simulink model "peacockElettricaSimulink"  (R2026a)
settings: Solver=FixedStepAuto  StopTime=40  FixedStep=0.001  EnableMultiTasking=on
InitFcn:
  | run('setupParams.m');
  | %run("tracks\track2.m");
StopFcn:
  | plot(out.X, out.Y);
  | axis equal;
  | grid on;
model workspace: external: MATLAB File (data not in the file)
values from neighbouring files (symbols this model uses):
  aero_bal_r = 0.5    [setupParams.m]    (also in setupParamsSingle.m)
  Af = 1.1    [setupParams.m]    (also in setupParamsSingle.m)
  auto_speed = 0    [setupParams.m]
  ay_limit = 15.0    (= 15)    [setupParams.m]    (also in setupParamsSingle.m)
  brake_bias_f = 0.40    (= 0.4)    [setupParams.m]    (also in setupParamsSingle.m = 0.6)
  brake_bias_r = 1 - brake_bias_f    (= 0.6)    [setupParams.m]    (also in setupParamsSingle.m = 0.4)
  camber_front = -1.5    [setupParams.m]    (also in setupParamsSingle.m)
  camber_rear = -1    [setupParams.m]    (also in setupParamsSingle.m)
  Cl = 1.0    (= 1)    [setupParams.m]    (also in setupParamsSingle.m)
  deathzone_APP = 5    [setupParams.m]    (also in setupParamsSingle.m)
  e_yaw_deadzone = 0.03    [setupParams.m]
  falling_slew_rate_torque = -500    [setupParams.m]    (also in setupParamsSingle.m)
  g = 9.81    [setupParams.m]    (also in setupParamsSingle.m)
  gnd_displ = 0.0    (= 0)    [setupParams.m]    (also in setupParamsSingle.m)
  h_o = 0.35    [setupParams.m]    (also in setupParamsSingle.m)
  I_charge_max = 21    [setupParams.m]
  I_discharge_max = 90    [setupParams.m]
  K_roll_rear = 0.6    [setupParams.m]    (also in setupParamsSingle.m = 0.5)
  Kus = 0.03    [setupParams.m]    (also in setupParamsSingle.m = 0)
  l_f = 0.775    [setupParams.m]    (also in setupParamsSingle.m)
  l_r = 0.775    [setupParams.m]    (also in setupParamsSingle.m)
  launch_ramp_rate = 1000.0    (= 1000)    [setupParams.m]    (also in setupParamsSingle.m)
  launch_V_thresh = 5.0    (= 5)    [setupParams.m]    (also in setupParamsSingle.m)
  mass = 320    [setupParams.m]    (also in setupParamsSingle.m = 300)
  mu = 1.5    [setupParams.m]    (also in setupParamsSingle.m)
  nominal_ramp_rate = 1000.0    (= 1000)    [setupParams.m]    (also in setupParamsSingle.m)
  overslip_factor = 1.01    [setupParams.m]    (also in setupParamsSingle.m = 1.13)
  pa_front_wheel = 82700    [setupParams.m]    (also in setupParamsSingle.m)
  pa_rear_wheel = 82700    [setupParams.m]    (also in setupParamsSingle.m)
  pedal_bp = (0:10:100)'    [setupParams.m]    (also in setupParamsSingle.m)
  pedal_map = (pedal_bp / 100) .^ pedal_alpha    [setupParams.m]    (also in setupParamsSingle.m = (pedal_bp / 100) .^ pedal_alpha.Value)
  R_wheel = 0.2032    [setupParams.m]    (also in setupParamsSingle.m)
  regen_I_cont_A = 14.0    (= 14)    [setupParams.m]    (also in setupParamsSingle.m)
  regen_I_peak_A = 21.0    (= 21)    [setupParams.m]    (also in setupParamsSingle.m)
  regen_I_peak_dur_s = 4.0    (= 4)    [setupParams.m]    (also in setupParamsSingle.m)
  regen_P_batt_max_W = 35000    [setupParams.m]    (also in setupParamsSingle.m)
  regen_pedal_thr = 5.0    (= 5)    [setupParams.m]    (also in setupParamsSingle.m = 10)
  regen_speed_crit_rpm = 1000    [setupParams.m]    (also in setupParamsSingle.m = 500)
  regen_speed_min_rpm = 4000    [setupParams.m]    (also in setupParamsSingle.m = 3000)
  regen_T_max = 9    [setupParams.m]    (also in setupParamsSingle.m = Simulink.Parameter(T_rated.Value/2))
  rho = 1.225    [setupParams.m]    (also in setupParamsSingle.m)
  rid_eff = 0.80    (= 0.8)    [setupParams.m]    (also in setupParamsSingle.m)
  rid_ratio = 15    [setupParams.m]    (also in setupParamsSingle.m)
  rising_slew_rate_torque = 100    [setupParams.m]    (also in setupParamsSingle.m)
  rpm_safe_threshold = 100    [setupParams.m]
  scale_factor_front = ones(27, 1)    [setupParams.m]    (also in setupParamsSingle.m)
  scale_factor_rear = ones(27, 1)    [setupParams.m]    (also in setupParamsSingle.m)
  slip_bc_coeff = 10    [setupParams.m]    (also in setupParamsSingle.m = Simulink.Parameter(1.5))
  slip_filt_N = 80    [setupParams.m]    (also in setupParamsSingle.m = 15)
  slip_Kd = 0.8    [setupParams.m]    (also in setupParamsSingle.m = Simulink.Parameter(5.0))
  slip_Ki = 13.0    (= 13)    [setupParams.m]    (also in setupParamsSingle.m = Simulink.Parameter(110.0))
  slip_Kp = 50.0    (= 50)    [setupParams.m]    (also in setupParamsSingle.m = Simulink.Parameter(180.0))
  slip_low_sat = 0.0    (= 0)    [setupParams.m]    (also in setupParamsSingle.m)
  slip_ref = 0.15    [setupParams.m]    (also in setupParamsSingle.m = Simulink.Parameter(0.15))
  slip_up_sat = 25    [setupParams.m]    (also in setupParamsSingle.m = 21)
  slip_V_min = 3    [setupParams.m]    (also in setupParamsSingle.m = 1)
  steer_ratio = 4.2    [pure_pursuit.m]    (also in setupParams.m; setupParamsSingle.m)
  steering_deadband = 1    [setupParams.m]
  T_headroom_k = 13.0    (= 13)    [setupParams.m]    (also in setupParamsSingle.m = Simulink.Parameter(5.0))
  T_headroom_max = 9    [setupParams.m]    (also in setupParamsSingle.m = Simulink.Parameter(5.0))
  T_peak = 20    [setupParams.m]    (also in setupParamsSingle.m = 21)
  T_rated = 9.8    [setupParams.m]    (also in setupParamsSingle.m = Simulink.Parameter(9.8))
  track_width = (track_width_r + track_width_f)/2    (= 1.2)    [setupParams.m]    (also in setupParamsSingle.m = sqrt(track_width_r^2 + track_width_f^2))
  track_width_f = 1.2    [setupParams.m]    (also in setupParamsSingle.m)
  track_width_r = 1.2    [setupParams.m]    (also in setupParamsSingle.m)
  Ts = 0.01    [setupParams.m]    (also in setupParamsSingle.m)
  tvc_bc = 17    [setupParams.m]
  tvc_D_thresh = 0.060    (= 0.06)    [setupParams.m]    (also in setupParamsSingle.m)
  tvc_D_thresh_off = 0.03    [setupParams.m]    (also in setupParamsSingle.m)
  tvc_Kd = 100    [setupParams.m]    (also in setupParamsSingle.m = Simulink.Parameter(5))
  tvc_Ki = 150    [setupParams.m]    (also in setupParamsSingle.m = Simulink.Parameter(10))
  tvc_Kp = 650    [setupParams.m]    (also in setupParamsSingle.m = Simulink.Parameter(70))
  tvc_N_filter = 25    [setupParams.m]    (also in setupParamsSingle.m = Simulink.Parameter(20))
  tvc_sat_dMz = 700    [setupParams.m]    (also in setupParamsSingle.m = Simulink.Parameter(10.0))
  tvc_throttle_on = 3.0    (= 3)    [setupParams.m]    (also in setupParamsSingle.m = Simulink.Parameter(3.0))
  tvc_tr = 5    [setupParams.m]    (also in setupParamsSingle.m = Simulink.Parameter(1.0))
  tvc_V_off = 2.0    (= 2)    [setupParams.m]    (also in setupParamsSingle.m = Simulink.Parameter(2.0))
  tvc_V_on = 4.0    (= 4)    [setupParams.m]    (also in setupParamsSingle.m = Simulink.Parameter(4.0))
  tvc_yaw_thresh = 0.08    [setupParams.m]    (also in setupParamsSingle.m)
  tvc_yaw_thresh_off = 0.04    [setupParams.m]    (also in setupParamsSingle.m)
  V_dc = 540    [setupParams.m]    (also in setupParamsSingle.m)
  w_engine = 0.005    [setupParams.m]    (also in setupParamsSingle.m)
  wheelbase = l_f + l_r    (= 1.55)    [setupParams.m]    (also in setupParamsSingle.m)
undefined symbols (not defined in the file or in its folder): V_ref, X_ref, Y_ref
libraries: simulink x74, slpidlib x8, vehdynlibtire x8, dspsigops x4, vehdynlibsteering x2, autolibshared x2, sim3dautolib x2, sim3dlib x1, robotalgslib x1
(part 4 of 6)

== system peacockElettricaSimulink/DriveController_/MTFC ==
  note: Minimum Torque Follower Controller
      | (derating)
  Throttle : Inport
  Derating_RL : Inport  Port=2
  Derating_RR : Inport  Port=3
  Constant : Constant  Value=T_peak
  Constant1 : Constant  Value=T_rated
  Gain : Gain  Gain=T_peak*0.01
  Logical Operator : Logic  Operator=OR  AllPortsSameDT=off  OutDataTypeStr=boolean
  Min : MinMax  Inputs=2
  Rate Limiter : RateLimiter  RisingSlewLimit=250  FallingSlewLimit=-250  SampleTimeMode=inherited
  Rate Limiter1 : RateLimiter  RisingSlewLimit=250  FallingSlewLimit=-10  SampleTimeMode=inherited
  Switch : Switch  Criteria=u2 > Threshold  Threshold=0.5  SaturateOnIntegerOverflow=off  InputSameDT=off
  T_req_MTFC : Outport
  wires:
  Min/1 -> Rate Limiter1/1  "out"
  Derating_RL/1 -> Logical Operator/1
  Logical Operator/1 -> Switch/2  "or"
  Derating_RR/1 -> Logical Operator/2
  Throttle/1 -> Gain/1
  Constant1/1 -> Switch/1  "rated"
  Constant/1 -> Switch/3  "peak"
  Switch/1 -> Rate Limiter/1
  Gain/1 -> Min/1  "req"
  Rate Limiter/1 -> Min/2  "T_lim_HW"
  Rate Limiter1/1 -> T_req_MTFC/1  "T_lim_HW"

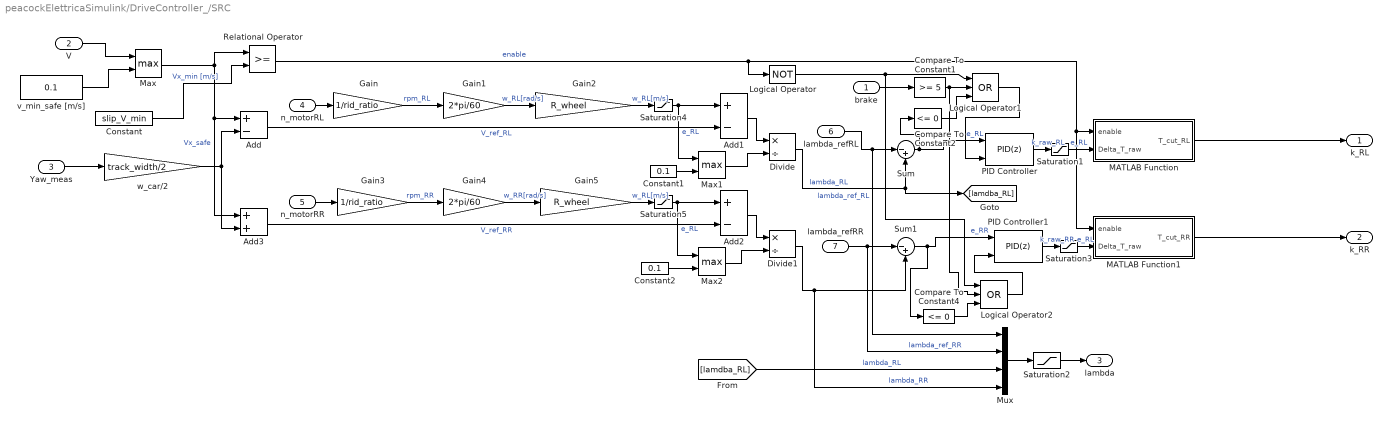
== system peacockElettricaSimulink/DriveController_/SRC ==
  brake : Inport
  V : Inport  Port=2
  Yaw_meas : Inport  Port=3
  n_motorRL : Inport  Port=4
  n_motorRR : Inport  Port=5
  lambda_refRL : Inport  Port=6
  lambda_refRR : Inport  Port=7
  Add : Sum  Inputs=+-
  Add1 : Sum  Inputs=+-
  Add2 : Sum  Inputs=+-
  Add3 : Sum
  Compare To Constant1 : simulink/Logic and Bit Operations/Compare To Constant  relop=>=  const=5  OutDataTypeStr=boolean
  Compare To Constant2 : simulink/Logic and Bit Operations/Compare To Constant  relop=<=  const=0  OutDataTypeStr=boolean
  Compare To Constant4 : simulink/Logic and Bit Operations/Compare To Constant  relop=<=  const=0  OutDataTypeStr=boolean
  Constant : Constant  Value=slip_V_min
  Constant1 : Constant  Value=0.1
  Constant2 : Constant  Value=0.1
  Divide : Product  Inputs=*/
  Divide1 : Product  Inputs=*/
  Gain : Gain  Gain=1/rid_ratio
  Gain1 : Gain  Gain=2*pi/60
  Gain2 : Gain  Gain=R_wheel
  Gain3 : Gain  Gain=1/rid_ratio
  Gain4 : Gain  Gain=2*pi/60
  Gain5 : Gain  Gain=R_wheel
  Logical Operator : Logic  Operator=NOT  AllPortsSameDT=off  OutDataTypeStr=boolean
  Logical Operator1 : Logic  Operator=OR  Inputs=3  AllPortsSameDT=off  OutDataTypeStr=boolean
  Logical Operator2 : Logic  Operator=OR  Inputs=3  AllPortsSameDT=off  OutDataTypeStr=boolean
  MATLAB Function : MATLAB Function  TreatAsAtomicUnit=on
  MATLAB Function1 : MATLAB Function  TreatAsAtomicUnit=on
  Max : MinMax  Function=max  Inputs=2
  Max1 : MinMax  Function=max  Inputs=2
  Max2 : MinMax  Function=max  Inputs=2
  Mux : Mux
  PID Controller : slpidlib/PID Controller  Controller=PID  Form=Parallel  TimeDomain=Discrete-time  UseExternalTs=off  SampleTime=Ts  IntegratorMethod=Forward Euler  FilterMethod=Forward Euler  ControllerParametersSource=internal  P=slip_Kp  I=slip_Ki  UseKiTs=off  D=slip_Kd  UseExternalDerivativeSource=off  N=slip_filt_N  UseFilter=on  TunerSelectOption=Transfer Function Based (PID Tuner App)  InitialConditionSource=internal  InitialConditionForIntegrator=0  InitialConditionForFilter=0  DifferentiatorICPrevScaledInput=0  ExternalReset=level  TrackingMode=off  Kt=1  LimitOutput=on  SatLimitsSource=internal  UpperSaturationLimit=slip_up_sat  LowerSaturationLimit=slip_low_sat  LinearizeAsGain=on  AntiWindupMode=back-calculation  Kb=slip_bc_coeff  LimitIntegrator=on  UpperIntegratorSaturationLimit=slip_up_sat  LowerIntegratorSaturationLimit=slip_low_sat  POutMin=[]  POutMax=[]  IOutMin=[]  IOutMax=[]  DOutMin=[]  DOutMax=[]  NOutMin=[]  NOutMax=[]  SumOutMin=[]  SumOutMax=[]  SaturationOutMin=[]  SaturationOutMax=[]  PParamMin=[]  PParamMax=[]  IParamMin=[]  IParamMax=[]  DParamMin=[]  DParamMax=[]  NParamMin=[]  NParamMax=[]  KbParamMin=[]  KbParamMax=[]  KtParamMin=[]  KtParamMax=[]  KbOutMin=[]  KbOutMax=[]  KtOutMin=[]  KtOutMax=[]  IntegratorOutMin=[]  IntegratorOutMax=[]  FilterOutMin=[]  FilterOutMax=[]  SumI1OutMin=[]  SumI1OutMax=[]  SumI2OutMin=[]  SumI2OutMax=[]  SumI3OutMin=[]  SumI3OutMax=[]  SumI4OutMin=[]  SumI4OutMax=[]  SumDOutMin=[]  SumDOutMax=[]  DifferentiatorOutMin=[]  DifferentiatorOutMax=[]  FilterDiffOutCoefMin=[]  FilterDiffOutCoefMax=[]  ReciprocalOutMin=[]  ReciprocalOutMax=[]  SumDenOutMin=[]  SumDenOutMax=[]  SumNumOutMin=[]  SumNumOutMax=[]  DivideOutMin=[]  DivideOutMax=[]  UdiffTsProdOutMin=[]  UdiffTsProdOutMax=[]  NTsProdOutMin=[]  NTsProdOutMax=[]  UintegralTsProdOutMin=[]  UintegralTsProdOutMax=[]  UngainTsProdOutMin=[]  UngainTsProdOutMax=[]  ClampingZeroOutDataTypeStr=Inherit: Inherit via back propagation  ClampingZeroOutMin=[]  ClampingZeroOutMax=[]  FilterDenConstantOutDataTypeStr=Inherit: Inherit via back propagation  FilterDenConstantOutMin=[]  FilterDenConstantOutMax=[]  PCopyOutDataTypeStr=Inherit: Inherit via back propagation  PCopyOutMin=[]  PCopyOutMax=[]  NCopyOutDataTypeStr=Inherit: Inherit via back propagation  NCopyOutMin=[]  NCopyOutMax=[]  IntegratorContinuousStateAttributes=''  IntegratorStateMustResolveToSignalObject=off  IntegratorRTWStateStorageClass=Auto  FilterContinuousStateAttributes=''  FilterStateMustResolveToSignalObject=off  FilterRTWStateStorageClass=Auto  ParallelPVariant=InternalParameters  IdealPVariant=Disabled  IVariant=InternalParameters  DVariant=InternalParameters  IntegratorVariant=Discrete  SatVariant=Enabled  AWVariant=BackCalculation  PCopyVariant=Disabled  TRVariant=Disabled  FdbkBlocksVariant=Forward  IdealPFdbkVariant=Disabled  SatFdbkVariant=Disabled  DerivativeFilterVariant=ForwardEulerFilter  NVariant=InternalParameters  NCopyVariant=Disabled  FilterICVariant=InternalICsFilter  IntegratorICVariant=InternalICs  ExternalResetVariant=ExternalReset  TRSumVariant=Passthrough  SumFdbkVariant=Disabled  SumVariant=Sum_PID  TsampFilterVariant=InternalTs  TsampNgainVariant=Passthrough  TsampIntegralVariant=Disabled_SignalSpec  ExternalSaturationOutDataTypeStr=Inherit: Same as second input  DerivativeSourceVariant=ErrorSignal  PreIntVariant=InternalPreInt
  PID Controller1 : slpidlib/PID Controller  Controller=PID  Form=Parallel  TimeDomain=Discrete-time  UseExternalTs=off  SampleTime=Ts  IntegratorMethod=Forward Euler  FilterMethod=Forward Euler  ControllerParametersSource=internal  P=slip_Kp  I=slip_Ki  UseKiTs=off  D=slip_Kd  UseExternalDerivativeSource=off  N=slip_filt_N  UseFilter=on  TunerSelectOption=Transfer Function Based (PID Tuner App)  InitialConditionSource=internal  InitialConditionForIntegrator=0  InitialConditionForFilter=0  DifferentiatorICPrevScaledInput=0  ExternalReset=level  TrackingMode=off  Kt=1  LimitOutput=on  SatLimitsSource=internal  UpperSaturationLimit=slip_up_sat  LowerSaturationLimit=slip_low_sat  LinearizeAsGain=on  AntiWindupMode=back-calculation  Kb=slip_bc_coeff  LimitIntegrator=on  UpperIntegratorSaturationLimit=slip_up_sat  LowerIntegratorSaturationLimit=slip_low_sat  POutMin=[]  POutMax=[]  IOutMin=[]  IOutMax=[]  DOutMin=[]  DOutMax=[]  NOutMin=[]  NOutMax=[]  SumOutMin=[]  SumOutMax=[]  SaturationOutMin=[]  SaturationOutMax=[]  PParamMin=[]  PParamMax=[]  IParamMin=[]  IParamMax=[]  DParamMin=[]  DParamMax=[]  NParamMin=[]  NParamMax=[]  KbParamMin=[]  KbParamMax=[]  KtParamMin=[]  KtParamMax=[]  KbOutMin=[]  KbOutMax=[]  KtOutMin=[]  KtOutMax=[]  IntegratorOutMin=[]  IntegratorOutMax=[]  FilterOutMin=[]  FilterOutMax=[]  SumI1OutMin=[]  SumI1OutMax=[]  SumI2OutMin=[]  SumI2OutMax=[]  SumI3OutMin=[]  SumI3OutMax=[]  SumI4OutMin=[]  SumI4OutMax=[]  SumDOutMin=[]  SumDOutMax=[]  DifferentiatorOutMin=[]  DifferentiatorOutMax=[]  FilterDiffOutCoefMin=[]  FilterDiffOutCoefMax=[]  ReciprocalOutMin=[]  ReciprocalOutMax=[]  SumDenOutMin=[]  SumDenOutMax=[]  SumNumOutMin=[]  SumNumOutMax=[]  DivideOutMin=[]  DivideOutMax=[]  UdiffTsProdOutMin=[]  UdiffTsProdOutMax=[]  NTsProdOutMin=[]  NTsProdOutMax=[]  UintegralTsProdOutMin=[]  UintegralTsProdOutMax=[]  UngainTsProdOutMin=[]  UngainTsProdOutMax=[]  ClampingZeroOutDataTypeStr=Inherit: Inherit via back propagation  ClampingZeroOutMin=[]  ClampingZeroOutMax=[]  FilterDenConstantOutDataTypeStr=Inherit: Inherit via back propagation  FilterDenConstantOutMin=[]  FilterDenConstantOutMax=[]  PCopyOutDataTypeStr=Inherit: Inherit via back propagation  PCopyOutMin=[]  PCopyOutMax=[]  NCopyOutDataTypeStr=Inherit: Inherit via back propagation  NCopyOutMin=[]  NCopyOutMax=[]  IntegratorContinuousStateAttributes=''  IntegratorStateMustResolveToSignalObject=off  IntegratorRTWStateStorageClass=Auto  FilterContinuousStateAttributes=''  FilterStateMustResolveToSignalObject=off  FilterRTWStateStorageClass=Auto  ParallelPVariant=InternalParameters  IdealPVariant=Disabled  IVariant=InternalParameters  DVariant=InternalParameters  IntegratorVariant=Discrete  SatVariant=Enabled  AWVariant=BackCalculation  PCopyVariant=Disabled  TRVariant=Disabled  FdbkBlocksVariant=Forward  IdealPFdbkVariant=Disabled  SatFdbkVariant=Disabled  DerivativeFilterVariant=ForwardEulerFilter  NVariant=InternalParameters  NCopyVariant=Disabled  FilterICVariant=InternalICsFilter  IntegratorICVariant=InternalICs  ExternalResetVariant=ExternalReset  TRSumVariant=Passthrough  SumFdbkVariant=Disabled  SumVariant=Sum_PID  TsampFilterVariant=InternalTs  TsampNgainVariant=Passthrough  TsampIntegralVariant=Disabled_SignalSpec  ExternalSaturationOutDataTypeStr=Inherit: Same as second input  DerivativeSourceVariant=ErrorSignal  PreIntVariant=InternalPreInt
  Relational Operator : RelationalOperator  OutDataTypeStr=boolean  RndMeth=Simplest  InputSameDT=off
  Saturation1 : Saturate  UpperLimit=inf  LowerLimit=-2
  Saturation2 : Saturate  UpperLimit=1  LowerLimit=0
  Saturation3 : Saturate  UpperLimit=inf  LowerLimit=-2
  Saturation4 : Saturate  UpperLimit=inf  LowerLimit=0
  Saturation5 : Saturate  UpperLimit=inf  LowerLimit=0
  Sum : Sum  Inputs=|-+
  Sum1 : Sum  Inputs=|-+
  v_min_safe [m/s] : Constant  Value=0.1
  w_car/2 : Gain  Gain=track_width/2
  k_RL : Outport
  k_RR : Outport  Port=2
  lambda : Outport  Port=3
  wires:
  V/1 -> Max/1
  v_min_safe [m/s]/1 -> Max/2
  Max/1 -> Relational Operator/1, Add3/1, Add/1  "Vx_safe"
  Constant/1 -> Relational Operator/2  "Vx_min [m/s]"
  Yaw_meas/1 -> w_car/2/1
  Add/1 -> Add1/2  "V_ref_RL"
  n_motorRL/1 -> Gain/1
  Gain/1 -> Gain1/1  "rpm_RL"
  Add1/1 -> Divide/1
  Divide/1 -> [lamdba_RL], Sum/2  "lambda_RL"
  w_car/2/1 -> Add3/2, Add/2
  Gain1/1 -> Gain2/1  "w_RL[rad/s]"
  Gain2/1 -> Saturation4/1  "w_RL[m/s]"
  Gain4/1 -> Gain5/1  "w_RR[rad/s]"
  Gain3/1 -> Gain4/1  "rpm_RR"
  Divide1/1 -> Sum1/2, Mux/4  "lambda_RR"
  n_motorRR/1 -> Gain3/1
  Add3/1 -> Add2/2  "V_ref_RR"
  Add2/1 -> Divide1/1
  Relational Operator/1 -> MATLAB Function1/1(enable), MATLAB Function/1(enable), Logical Operator/1  "enable"
  PID Controller/1 -> Saturation1/1  "k_raw_RL"
  MATLAB Function/1(T_cut_RL) -> k_RL/1
  PID Controller1/1 -> Saturation3/1  "k_raw_RR"
  lambda_refRR/1 -> Mux/2, Sum1/1  "lambda_ref_RR"
  MATLAB Function1/1(T_cut_RR) -> k_RR/1
  Sum1/1 -> Compare To Constant4/1, PID Controller1/1  "e_RR"
  Sum/1 -> PID Controller/1, Compare To Constant2/1  "e_RL"
  Max1/1 -> Divide/2
  Constant1/1 -> Max1/2
  Max2/1 -> Divide1/2
  Constant2/1 -> Max2/2
  Gain5/1 -> Saturation5/1  "w_RL[m/s]"
  Mux/1 -> Saturation2/1
  Saturation2/1 -> lambda/1
  Saturation1/1 -> MATLAB Function/2(Delta_T_raw)  "e_RL"
  Saturation3/1 -> MATLAB Function1/2(Delta_T_raw)  "e_RL"
  Logical Operator1/1 -> PID Controller/2
  [lamdba_RL] -> Mux/3  "lambda_RL"
  Saturation4/1 -> Max1/1, Add1/1  "e_RL"
  Saturation5/1 -> Max2/1, Add2/1  "e_RL"
  Logical Operator/1 -> Logical Operator2/1, Logical Operator1/1
  Compare To Constant2/1 -> Logical Operator1/3
  Compare To Constant4/1 -> Logical Operator2/3
  lambda_refRL/1 -> Mux/1, Sum/1  "lambda_ref_RL"
  Logical Operator2/1 -> PID Controller1/2
  brake/1 -> Compare To Constant1/1
  Compare To Constant1/1 -> Logical Operator2/2, Logical Operator1/2

== system peacockElettricaSimulink/DriveController_/TVC ==
  note: Momento Imbardata di correzione
  T_req : Inport
  e_yaw : Inport  Port=2
  T_RL_act : Inport  Port=3
  T_RR_act : Inport  Port=4
  n_motorRL : Inport  Port=5
  n_motorRR : Inport  Port=6
  D : Inport  Port=7
  w_slip : Inport  Port=8
  T_max_RL : Inport  Port=9
  T_max_RR : Inport  Port=10
  1-D Lookup Table : Lookup_n-D  NumberOfTableDimensions=1  BreakpointsForDimension1=[0,steering_deadband,5]  Table=[0,0,1]  ExtrapMethod=Clip  UseLastTableValue=on  InternalRulePriority=Speed  RndMeth=Simplest
  Abs1 : Abs  SaturateOnIntegerOverflow=off
  Compare To Constant3 : simulink/Logic and Bit Operations/Compare To Constant  relop===  const=0  OutDataTypeStr=boolean
  Constant : Constant  Value=0
  Dead Zone : DeadZone  LowerValue=-e_yaw_deadzone  UpperValue=e_yaw_deadzone
  Gain : Gain  Gain=180*steer_ratio/pi
  MATLAB Function : MATLAB Function  TreatAsAtomicUnit=on
  MATLAB Function1 : MATLAB Function  TreatAsAtomicUnit=on
  Memory : Memory
  PID Controller : slpidlib/PID Controller  Controller=PID  Form=Parallel  TimeDomain=Discrete-time  UseExternalTs=off  SampleTime=Ts  IntegratorMethod=Forward Euler  FilterMethod=Forward Euler  ControllerParametersSource=internal  P=tvc_Kp  I=tvc_Ki  UseKiTs=off  D=tvc_Kd  UseExternalDerivativeSource=off  N=tvc_N_filter  UseFilter=on  TunerSelectOption=Transfer Function Based (PID Tuner App)  InitialConditionSource=external  InitialConditionForIntegrator=0  InitialConditionForFilter=0  DifferentiatorICPrevScaledInput=0  ExternalReset=level  TrackingMode=on  Kt=tvc_tr  LimitOutput=on  SatLimitsSource=internal  UpperSaturationLimit=tvc_sat_dMz  LowerSaturationLimit=-tvc_sat_dMz  LinearizeAsGain=on  AntiWindupMode=back-calculation  Kb=tvc_bc  LimitIntegrator=off  UpperIntegratorSaturationLimit=inf  LowerIntegratorSaturationLimit=-inf  POutMin=[]  POutMax=[]  IOutMin=[]  IOutMax=[]  DOutMin=[]  DOutMax=[]  NOutMin=[]  NOutMax=[]  SumOutMin=[]  SumOutMax=[]  SaturationOutMin=[]  SaturationOutMax=[]  PParamMin=[]  PParamMax=[]  IParamMin=[]  IParamMax=[]  DParamMin=[]  DParamMax=[]  NParamMin=[]  NParamMax=[]  KbParamMin=[]  KbParamMax=[]  KtParamMin=[]  KtParamMax=[]  KbOutMin=[]  KbOutMax=[]  KtOutMin=[]  KtOutMax=[]  IntegratorOutMin=[]  IntegratorOutMax=[]  FilterOutMin=[]  FilterOutMax=[]  SumI1OutMin=[]  SumI1OutMax=[]  SumI2OutMin=[]  SumI2OutMax=[]  SumI3OutMin=[]  SumI3OutMax=[]  SumI4OutMin=[]  SumI4OutMax=[]  SumDOutMin=[]  SumDOutMax=[]  DifferentiatorOutMin=[]  DifferentiatorOutMax=[]  FilterDiffOutCoefMin=[]  FilterDiffOutCoefMax=[]  ReciprocalOutMin=[]  ReciprocalOutMax=[]  SumDenOutMin=[]  SumDenOutMax=[]  SumNumOutMin=[]  SumNumOutMax=[]  DivideOutMin=[]  DivideOutMax=[]  UdiffTsProdOutMin=[]  UdiffTsProdOutMax=[]  NTsProdOutMin=[]  NTsProdOutMax=[]  UintegralTsProdOutMin=[]  UintegralTsProdOutMax=[]  UngainTsProdOutMin=[]  UngainTsProdOutMax=[]  ClampingZeroOutDataTypeStr=Inherit: Inherit via back propagation  ClampingZeroOutMin=[]  ClampingZeroOutMax=[]  FilterDenConstantOutDataTypeStr=Inherit: Inherit via back propagation  FilterDenConstantOutMin=[]  FilterDenConstantOutMax=[]  PCopyOutDataTypeStr=Inherit: Inherit via back propagation  PCopyOutMin=[]  PCopyOutMax=[]  NCopyOutDataTypeStr=Inherit: Inherit via back propagation  NCopyOutMin=[]  NCopyOutMax=[]  IntegratorContinuousStateAttributes=''  IntegratorStateMustResolveToSignalObject=off  IntegratorRTWStateStorageClass=Auto  FilterContinuousStateAttributes=''  FilterStateMustResolveToSignalObject=off  FilterRTWStateStorageClass=Auto  ParallelPVariant=InternalParameters  IdealPVariant=Disabled  IVariant=InternalParameters  DVariant=InternalParameters  IntegratorVariant=Discrete  SatVariant=Enabled  AWVariant=BackCalculation  PCopyVariant=Disabled  TRVariant=Enabled  FdbkBlocksVariant=Forward  IdealPFdbkVariant=Disabled  SatFdbkVariant=Disabled  DerivativeFilterVariant=ForwardEulerFilter  NVariant=InternalParameters  NCopyVariant=Disabled  FilterICVariant=ExternalICs  IntegratorICVariant=ExternalICs  ExternalResetVariant=ExternalReset  TRSumVariant=TrackingMode  SumFdbkVariant=Disabled  SumVariant=Sum_PID  TsampFilterVariant=InternalTs  TsampNgainVariant=Passthrough  TsampIntegralVariant=Disabled_SignalSpec  ExternalSaturationOutDataTypeStr=Inherit: Same as second input  DerivativeSourceVariant=ErrorSignal  PreIntVariant=InternalPreInt
  Product : Product  Inputs=3
  Scope : Scope  NumInputPorts=3
      settings: ActiveDisplayYMinimum=-0.17006762266637193  ActiveDisplayYMaximum=0.69301535210007792
  Sum3 : Sum  Inputs=|-+
  TorqueAllocator : MATLAB Function  TreatAsAtomicUnit=on  SystemSampleTime=0.05
  T_TVC_RL : Outport
  T_TVC_RR : Outport  Port=2
  wires:
  PID Controller/1 -> MATLAB Function/1(dMz)  "dMz"
  Sum3/1 -> MATLAB Function1/1(dT_act)  "dT_act"
  MATLAB Function1/1(dMz_act) -> PID Controller/5, Memory/1  "dMz_act"
  T_RL_act/1 -> Sum3/1
  T_RR_act/1 -> Sum3/2
  Product/1 -> Scope/3, TorqueAllocator/2(dT)  "dT_real"
  TorqueAllocator/1(T_RL_cmd) -> T_TVC_RL/1
  TorqueAllocator/2(T_RR_cmd) -> T_TVC_RR/1
  n_motorRL/1 -> TorqueAllocator/3(n_motorRL)
  n_motorRR/1 -> TorqueAllocator/4(n_motorRR)
  Constant/1 -> PID Controller/4
  Memory/1 -> PID Controller/3
  e_yaw/1 -> Scope/1, Dead Zone/1
  D/1 -> TorqueAllocator/5(D), Gain/1  "D_rad"
  T_req/1 -> TorqueAllocator/1(T_req)
  Gain/1 -> Abs1/1  "steering°"
  MATLAB Function/1(dT) -> Scope/2, Product/1  "dT_pi"
  1-D Lookup Table/1 -> Product/3
  Abs1/1 -> 1-D Lookup Table/1
  w_slip/1 -> Product/2
  T_max_RL/1 -> TorqueAllocator/6(T_grip_max_RL)
  T_max_RR/1 -> TorqueAllocator/7(T_grip_max_RR)
  Dead Zone/1 -> Compare To Constant3/1, PID Controller/1
  Compare To Constant3/1 -> PID Controller/2

== system peacockElettricaSimulink/DriveController_/Yaw_th ==
  V : Inport
  D_rad : Inport  Port=2
  Bicycle Model Dynamic : MATLAB Function  TreatAsAtomicUnit=on
  Rate Lmiter : RateLimiter  SampleTimeMode=inherited
  Trigonometric Function : Trigonometry  Operator=tan
  tand safe : MATLAB Function  TreatAsAtomicUnit=on
  yaw_saturation : MATLAB Function  TreatAsAtomicUnit=on
  yaw_th : Outport
  wires:
  tand safe/1(tand_safe) -> Bicycle Model Dynamic/2(tan_delta)  "tan delta"
  Trigonometric Function/1 -> tand safe/1(tand)
  Bicycle Model Dynamic/1(yaw_th) -> Rate Lmiter/1  "yaw_th"
  V/1 -> Bicycle Model Dynamic/1(V), yaw_saturation/2(V)  "V"
  D_rad/1 -> Trigonometric Function/1
  Rate Lmiter/1 -> yaw_saturation/1(yaw_th)  "yaw_th"
  yaw_saturation/1(yaw_sat) -> yaw_th/1  "yaw_sat"

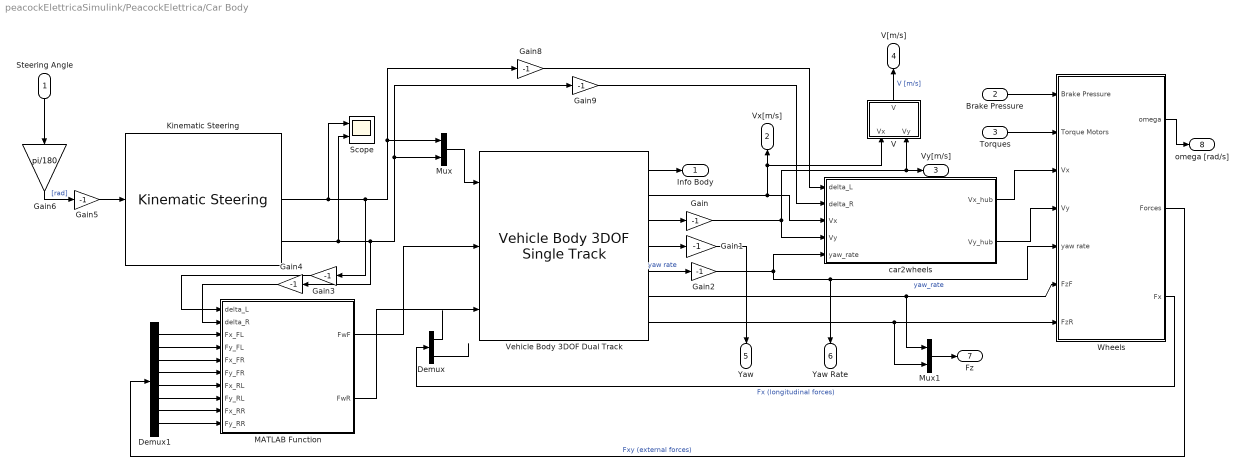
== system peacockElettricaSimulink/PeacockElettrica/Car Body ==
  Steering Angle : Inport
  Brake Pressure : Inport  Port=2
  Torques : Inport  Port=3
  Demux : Demux  Outputs=2
  Demux1 : Demux  Outputs=8
  Gain{,1..5,8..9} (8 alike) : Gain  Gain=-1
  Gain6 : Gain  Gain=pi/180
  Kinematic Steering : vehdynlibsteering/Kinematic Steering  StrgType=Ackerman  StrgRatioType=Constant  Loc=Front  NrmlFctr=0.01  TrckWdth=track_width  WhlBase=wheelbase  Db=0  StrgRng=pi  StrgAngBpts="[-6.2832   -5.0265   -3.7699   -2.5133   -1.2566         0    1.2566    2.5133    3.7699    5.0265    6.2832]"  StrgRatioTbl=|  StrgRatio=steer_ratio  PctAckIn=off  PctAck=100  PctAckTbl=ones(1,11)*100  StrgArmLngth=0.1  RckCsLngth=0.5  TieRodLngth=0.248  D=0.2  PnnRadius=0.00085818  PnnRadiusTbl="[0.0055    0.0055    0.0056    0.0057    0.0058    0.0057    0.0057    0.0057    0.0056    0.0055    0.0055]"  RodLngth=0.1  ParaArmLngth=0.9  aMode=2
      | [13.5000   13.3750   13.2500   13.1250   13.0000   13.0000   13.0000   13.1250   13.2500   13.3750   13.5000
      | ]
  MATLAB Function : MATLAB Function  TreatAsAtomicUnit=on
  Mux : Mux  Inputs=2
  Mux1 : Mux  Inputs=2
  Scope : Scope  NumInputPorts=2
      settings: ActiveDisplayYMinimum=-0.19369023585862366  ActiveDisplayYMaximum=0.062259490327338275
  V : MATLAB Function  TreatAsAtomicUnit=on
  Vehicle Body 3DOF Dual Track : autolibshared/Vehicle Body 3DOF Single Track  trackMode=Dual  inputMode=External forces  frontSteerMode=on  rearSteerMode=off  extFMode=off  htchFMode=off  extMMode=off  htchMMode=off  windMode=off  extTamb=off  muMode=off  extGndPlnElev=off  extGndPlnRoll=off  extGndPlnPitch=off  extGndPlnDCM=off  extXo=off  extxdoto=off  extYo=off  extydoto=off  extpsio=off  extro=off  aMode=2  NF=n_wheels_f  NR=n_wheels_r  m=mass  a=l_f  b=l_r  h=h_o  dh=1  hh=0.2  X_o=0  xdot_o=0  d=0  hl=0  w=[track_width_f,track_width_r]  CalphaMode=Constant  sigmaMode=on  sigma_f=.1  sigma_r=.1  Cy_f=12e3  Cy_r=11e3  Cy_f_data="[1.396121365092108e+04\t4.232462640127975e+04\t6.754894575573687e+04\t8.835784428391886e+04\t1.043551700699839e+05\t1.158335754468729e+05\t1.234691551560788e+05\t1.280575366661118e+05\t1.298126639907242e+05\t1.298126639907242e+05]"  alpha_f_brk=[-0.785, -0.628, -0.471, -0.314, -0.157, 0.000, 0.157, 0.314, 0.471, 0.628, 0.785]  Fz_f_brk="[500\t1.555555555555556e+03\t2.611111111111111e+03\t3.666666666666667e+03\t4.722222222222223e+03\t5.777777777777777e+03\t6.833333333333333e+03\t7.888888888888889e+03\t8.944444444444445e+03\t10000]"  Cy_r_data="[1.396121365092108e+04\t4.232462640127975e+04\t6.754894575573687e+04\t8.835784428391886e+04\t1.043551700699839e+05\t1.158335754468729e+05\t1.234691551560788e+05\t1.280575366661118e+05\t1.298126639907242e+05\t1.298126639907242e+05]"  alpha_r_brk=[-0.785, -0.628, -0.471, -0.314, -0.157, 0.000, 0.157, 0.314, 0.471, 0.628, 0.785]  Fz_r_brk="[500\t1.555555555555556e+03\t2.611111111111111e+03\t3.666666666666667e+03\t4.722222222222223e+03\t5.777777777777777e+03\t6.833333333333333e+03\t7.888888888888889e+03\t8.944444444444445e+03\t10000]"  Fznom=5000  Y_o=0  ydot_o=0  Izz=Izz  psi_o=0  r_o=0  Af=Af  Cd=Cd  Cl=Cl  Cpm=.1  beta_w=[0 0.01:0.01:0.3]  Cs=[0:0.03:0.9]  Cym=[0 1e-6:0.01:0.3]  Pabs=pressure  Tair=air_temp  g=g  mu=1  GndPlnRoll=0  GndPlnPitch=0  GndPlnElev=0  xdot_tol=.01  Fxtire_sat=7e4  Fytire_sat=7e4  longOff=0  latOff=0  vertOff=0  wrapAng=off
      settings: LibrarySourceBlock=vehdynlibeom/Vehicle Body 3DOF Dual Track
  Wheels : Subsystem
  car2wheels : MATLAB Function  TreatAsAtomicUnit=on
  Info Body : Outport
  Vx[m/s] : Outport  Port=2
  Vy[m/s] : Outport  Port=3
  V[m/s] : Outport  Port=4
  Yaw : Outport  Port=5
  Yaw Rate : Outport  Port=6
  Fz : Outport  Port=7
  omega [rad/s] : Outport  Port=8
  wires:
  Gain/1 -> V/2(Vy), Vy[m/s]/1, car2wheels/4(Vy)
  Demux1/2 -> MATLAB Function/4(Fy_FL)
  Vehicle Body 3DOF Dual Track/1 -> Info Body/1
  Vehicle Body 3DOF Dual Track/4 -> Gain1/1
  Gain2/1 -> car2wheels/5(yaw_rate), Yaw Rate/1, Wheels/5(yaw rate)  "yaw_rate"
  Demux1/5 -> MATLAB Function/7(Fx_RL)
  Vehicle Body 3DOF Dual Track/3 -> Gain/1
  Vehicle Body 3DOF Dual Track/2 -> V/1(Vx), Vx[m/s]/1, car2wheels/3(Vx)
  Wheels/1(omega) -> omega [rad/s]/1
  Vehicle Body 3DOF Dual Track/6 -> Mux1/1, Wheels/6(FzF)
  Demux1/7 -> MATLAB Function/9(Fx_RR)
  Demux1/8 -> MATLAB Function/10(Fy_RR)
  Vehicle Body 3DOF Dual Track/5 -> Gain2/1  "yaw rate"
  Demux1/6 -> MATLAB Function/8(Fy_RL)
  Demux1/4 -> MATLAB Function/6(Fy_FR)
  MATLAB Function/1(FwF) -> Vehicle Body 3DOF Dual Track/2
  Demux1/3 -> MATLAB Function/5(Fx_FR)
  car2wheels/2(Vy_hub) -> Wheels/4(Vy)
  Demux1/1 -> MATLAB Function/3(Fx_FL)
  Torques/1 -> Wheels/2(Torque Motors)
  Steering Angle/1 -> Gain6/1
  Vehicle Body 3DOF Dual Track/7 -> Mux1/2, Wheels/7(FzR)
  Wheels/2(Forces) -> Demux1/1  "Fxy (external forces)"
  MATLAB Function/2(FwR) -> Vehicle Body 3DOF Dual Track/3
  Gain5/1 -> Kinematic Steering/1
  Mux/1 -> Vehicle Body 3DOF Dual Track/1
  Brake Pressure/1 -> Wheels/1(Brake Pressure)
  Gain6/1 -> Gain5/1  "[rad]"
  car2wheels/1(Vx_hub) -> Wheels/3(Vx)
  Gain1/1 -> Yaw/1
  Kinematic Steering/2 -> Scope/1, Gain3/1, Gain8/1, Mux/1
  Kinematic Steering/3 -> Scope/2, Gain4/1, Gain9/1, Mux/2
  Gain3/1 -> MATLAB Function/1(delta_L)
  Gain4/1 -> MATLAB Function/2(delta_R)
  Gain8/1 -> car2wheels/1(delta_L)
  Gain9/1 -> car2wheels/2(delta_R)
  V/1(V) -> V[m/s]/1  "V [m/s]"
  Mux1/1 -> Fz/1
  Wheels/3(Fx) -> Demux/1  "Fx (longitudinal forces)"
  Demux/1 -> ?
  Demux/2 -> ?

== system peacockElettricaSimulink/PeacockElettrica/G_motor_RL ==
  T_req : Inport
  rpm_motor : Inport  Port=2
  1-D Lookup Table : Lookup_n-D  NumberOfTableDimensions=1  BreakpointsForDimension1=[0, 9268, 11586.6]  Table=[21, 21, 9.8]  InternalRulePriority=Speed  RndMeth=Simplest
  Constant : Constant  Value=V_dc
  Derating : MATLAB Function  TreatAsAtomicUnit=on
  Field weakening : MATLAB Function  TreatAsAtomicUnit=on
  Gain : Gain  Gain=1/0.26
  I_n ^2 : Constant  Value=1681
  Integrator : Integrator  LimitOutput=on  UpperSaturationLimit=11586.6  LowerSaturationLimit=0
  Math Function : Math  Operator=square
  Min : MinMax  Inputs=3
  Sum : Sum  Inputs=|+-
  Transfer Fcn : TransferFcn  Denominator=[w_engine 1]
  Unit Delay : UnitDelay  SampleTime=-1
  Unit Delay1 : UnitDelay  SampleTime=-1
  T_out : Outport
  derating : Outport  Port=2
  wires:
  Sum/1 -> Integrator/1
  I_n ^2/1 -> Sum/2
  Gain/1 -> Math Function/1  "I_req"
  Math Function/1 -> Sum/1
  Integrator/1 -> 1-D Lookup Table/1
  Min/1 -> Transfer Fcn/1
  Transfer Fcn/1 -> T_out/1
  1-D Lookup Table/1 -> Derating/1(T_thermal), Min/1  "T_thermal_limit"
  Derating/1(derating_out) -> Unit Delay1/1
  rpm_motor/1 -> Field weakening/1(rpm_motor)
  Field weakening/1(T_limit) -> Min/3
  T_req/1 -> Derating/2(T_req), Gain/1, Min/2
  Constant/1 -> Field weakening/2(V_dc)
  Unit Delay1/1 -> Derating/3(derating_prev), derating/1

== system peacockElettricaSimulink/PeacockElettrica/G_motor_RR ==
  T_req : Inport
  rpm_motor : Inport  Port=2
  1-D Lookup Table : Lookup_n-D  NumberOfTableDimensions=1  BreakpointsForDimension1=[0, 9268, 11586.6]  Table=[21, 21, 9.8]  InternalRulePriority=Speed  RndMeth=Simplest
  Constant : Constant  Value=V_dc
  Gain : Gain  Gain=1/0.26
  I_n ^2 : Constant  Value=1681
  Integrator : Integrator  LimitOutput=on  UpperSaturationLimit=11586.6  LowerSaturationLimit=0
  MATLAB Function : MATLAB Function  TreatAsAtomicUnit=on
  MATLAB Function1 : MATLAB Function  TreatAsAtomicUnit=on
  Math Function : Math  Operator=square
  Min : MinMax  Inputs=3
  Sum : Sum  Inputs=|+-
  Transfer Fcn : TransferFcn  Denominator=[w_engine 1]
  Unit Delay : UnitDelay  SampleTime=-1
  T_out : Outport
  derating : Outport  Port=2
  wires:
  Sum/1 -> Integrator/1
  Integrator/1 -> 1-D Lookup Table/1
  T_req/1 -> MATLAB Function/2(T_req), Gain/1, Min/2
  Math Function/1 -> Sum/1
  Transfer Fcn/1 -> T_out/1
  Gain/1 -> Math Function/1  "I_req"
  I_n ^2/1 -> Sum/2
  rpm_motor/1 -> MATLAB Function1/1(rpm_motor)
  MATLAB Function1/1(T_limit) -> Min/3
  1-D Lookup Table/1 -> MATLAB Function/1(T_thermal), Min/1  "T_thermal_limit"
  Min/1 -> Transfer Fcn/1
  Constant/1 -> MATLAB Function1/2(V_dc)
  MATLAB Function/1(derating_out) -> Unit Delay/1
  Unit Delay/1 -> MATLAB Function/3(derating_prev), derating/1
